simulink model "logExample"  (R2016b)
settings: Solver=FixedStepAuto  StartTime=0.0  StopTime=10.0  RelTol=1e-3
undefined symbols (not defined in the file or in its folder): RGBLED_COLOR_ENUM, RGBLED_MODE_ENUM
libraries: pixhawk_slib_sensors_actuators x2, pixhawk_slib_misc_utils x1, simulink x1
settings Model: Creator=pixhawk  LastModifiedBy=pixhawk
settings OptimizationCC: DefaultParameterBehavior=Inlined  InlineInvariantSignals=on  MaxStackSize=64
settings DebuggingCC: ParameterTunabilityLossMsg=error
settings HardwareCC: ProdBitPerPointer=32  ProdBitPerSizeT=32  ProdBitPerPtrDiffT=32  ProdLargestAtomicInteger=Long  ProdLargestAtomicFloat=Double  ProdWordSize=32  ProdHWDeviceType=ARM Compatible->ARM Cortex
settings RTWCC: SystemTargetFile=ert.tlc  HardwareBoard=Pixhawk PX4  TLCOptions="-aInlineSetEventsForThisBaseRateFcn=TLC_FALSE -aSuppressMultiTaskScheduler=TLC_FALSE  -aRateBasedStepFcn=0"  TemplateMakefile=ert_default_tmf  Description=Embedded Coder  GenerateReport=on  Toolchain=Pixhawk Toolchain  IncludeHyperlinkInReport=on  LaunchReport=on  GenerateTraceInfo=on  GenerateTraceReport=on  GenerateTraceReportSl=on  GenerateTraceReportSf=on  GenerateTraceReportEml=on
settings CodeAppCC: ForceParamTrailComments=on  IgnoreCustomStorageClasses=off  OperatorAnnotations=on  SimulinkDataObjDesc=on  SFDataObjDesc=on  MATLABFcnDesc=on  InsertBlockDesc=on  MATLABSourceComments=on
settings ERTTargetCC: InlinedParameterPlacement=NonHierarchical  ERTCustomFileTemplate=PX4_codertarget_file_process.tlc

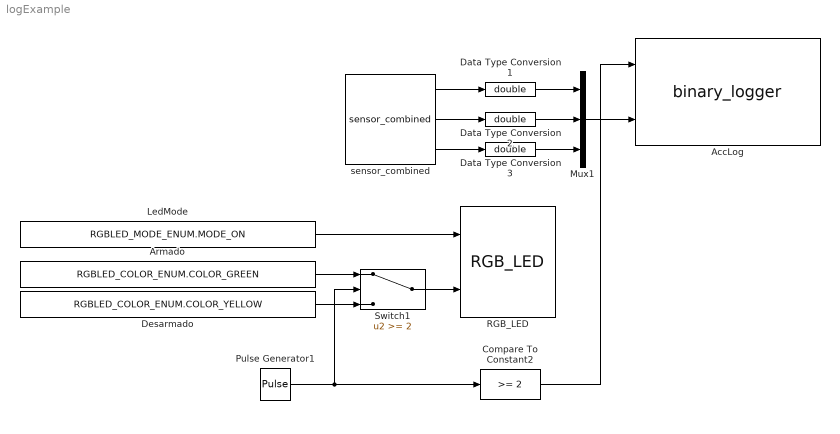
== system logExample ==
  AccLog : pixhawk_slib_misc_utils/binary_logger  logfile=/fs/microsd/log/logtest  cacheflag=off  numRecs=1000
  Armado : Constant  Value=RGBLED_COLOR_ENUM.COLOR_GREEN  OutDataTypeStr=Enum: RGBLED_COLOR_ENUM
  Compare To Constant2 : simulink/Logic and Bit Operations/Compare To Constant  relop=>=  const=2  OutDataTypeStr=boolean
  Data Type Conversion1 : DataTypeConversion  OutDataTypeStr=double
  Data Type Conversion2 : DataTypeConversion  OutDataTypeStr=double
  Data Type Conversion3 : DataTypeConversion  OutDataTypeStr=double
  Desarmado : Constant  Value=RGBLED_COLOR_ENUM.COLOR_YELLOW  OutDataTypeStr=Enum: RGBLED_COLOR_ENUM
  LedMode : Constant  Value=RGBLED_MODE_ENUM.MODE_ON  OutDataTypeStr=Enum: RGBLED_MODE_ENUM
  Mux1 : Mux  Inputs=3
  Pulse Generator1 : DiscretePulseGenerator  Amplitude=150  Period=1000  PulseWidth=700  SampleTime=0.004
  RGB_LED : pixhawk_slib_sensors_actuators/RGB_LED
  Switch1 : Switch  Threshold=2
  sensor_combined : pixhawk_slib_sensors_actuators/sensor_combined  sampletime=1/250  show_mag=off  show_acc=on  show_gyro=off  show_baro=off  show_ts=off
  wires:
  Switch1/1 -> RGB_LED/2
  Armado/1 -> Switch1/1
  Desarmado/1 -> Switch1/3
  LedMode/1 -> RGB_LED/1
  Pulse Generator1/1 -> Switch1/2, Compare To Constant2/1
  Mux1/1 -> AccLog/2
  Data Type Conversion1/1 -> Mux1/1
  Data Type Conversion2/1 -> Mux1/2
  Data Type Conversion3/1 -> Mux1/3
  sensor_combined/1 -> Data Type Conversion1/1
  sensor_combined/2 -> Data Type Conversion2/1
  sensor_combined/3 -> Data Type Conversion3/1
  Compare To Constant2/1 -> AccLog/1
